simulink model "symbolic_controller"  (Simulink 6.6)
settings: Solver=ode45  StartTime=0.0  StopTime=10.0  RelTol=1e-3
undefined symbols (not defined in the file): contr_name, uini
settings Model: Creator=manuelmazo  LastModifiedBy=manuelmazo  ExtModeAutoUpdateStatusClock=off

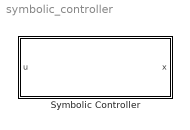
== system symbolic_controller ==
  "Symbolic Controller " : Subsystem  Orientation=left  mask{contr_name=contr_name, uini=uini}
      mask prompts: contr_name "Controller Name"; uini "Initial Controller State"
      mask init:
      | load(strcat(contr_name,'_symb'), 'params_symb');

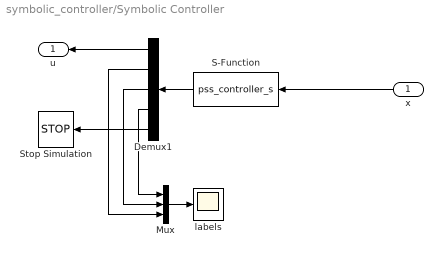
== system symbolic_controller/Symbolic Controller  ==
  x : Inport  Orientation=left
  Demux1 : Demux  Orientation=left  Outputs=5
  Mux : Mux  Inputs=3
  S-Function : S-Function  Orientation=left  FunctionName=pss_controller_s  Parameters=params_symb, contr_name, uini
  Stop Simulation : Stop  Orientation=left
  labels : Scope
  u : Outport  Orientation=left
  wires:
  S-Function/1 -> Demux1/1
  Demux1/4 -> Mux/1
  Demux1/3 -> Mux/2
  Demux1/2 -> Mux/3
  x/1 -> S-Function/1
  Demux1/1 -> u/1
  Demux1/5 -> Stop Simulation/1
  Mux/1 -> labels/1
